simulink model "DYN_03x"  (R2021a)
settings: Solver=FixedStepAuto  StartTime=0.0  StopTime=10  FixedStep=0.001  RelTol=1e-3
(part 1 of 9)
settings Model: Creator=TMP  LastModifiedBy=TMP
settings SolverCC: AlgebraicLoopSolver=TrustRegion
settings DebuggingCC: SFMachineParentedDataDiag=warning

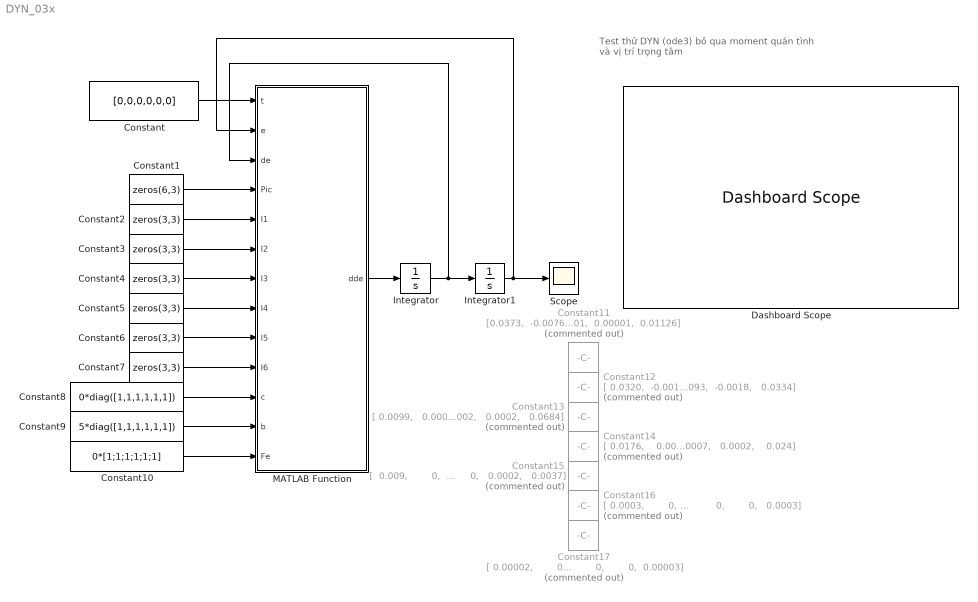
== system DYN_03x ==
  note: Test thử DYN (ode3)
      | bỏ qua moment quán tình và vị trí trọng tâm
  Constant : Constant  Value=[0,0,0,0,0,0]
  Constant1 : Constant  Value=zeros(6,3)
  Constant10 : Constant  Value=0*[1;1;1;1;1;1]
  Constant11 : Constant  Commented=on  Value=|
      | [0.0373,  -0.0076,   0.1064;
      |        0.1127,   0.0065,   0.0648;
      |        0.0447,   0.0125,  -0.0554;
      |        0.0006,   0.0052,   0.1068;
      |             0,   0.0062,   0.0195;
      |      -0.00001,  0.00001,  0.01126]
  Constant12 : Constant  Commented=on  Value=|
      | [ 0.0320,  -0.0017,   0.0093;
      |       -0.0017,   0.0364,  -0.0018;
      |        0.0093,  -0.0018,   0.0334]
  Constant13 : Constant  Commented=on  Value=|
      | [ 0.0099,   0.0008,  -0.0002;
      |        0.0008,   0.0646,   0.0002;
      |       -0.0002,   0.0002,   0.0684]
  Constant14 : Constant  Commented=on  Value=|
      | [ 0.0176,    0.001,   0.0007;
      |         0.001,   0.0195,   0.0002;
      |        0.0007,   0.0002,    0.024]
  Constant15 : Constant  Commented=on  Value=|
      | [  0.009,        0,        0;
      |             0,   0.0081,   0.0002;
      |             0,   0.0002,   0.0037]
  Constant16 : Constant  Commented=on  Value=|
      | [ 0.0003,        0,        0;
      |             0,   0.0002,        0;
      |             0,        0,   0.0003]
  Constant17 : Constant  Commented=on  Value=|
      | [ 0.00002,        0,        0;
      |              0,  0.00002,        0;
      |              0,        0,  0.00003]
  Constant{2..7} (6 alike) : Constant  Value=zeros(3,3)
  Constant8 : Constant  Value=0*diag([1,1,1,1,1,1])
  Constant9 : Constant  Value=5*diag([1,1,1,1,1,1])
  Dashboard Scope : DashboardScope
  Integrator : Integrator  InitialCondition=[0;0;0;0;0;0]
  Integrator1 : Integrator  InitialCondition=[0;0;0;0;0;0]
  MATLAB Function : MATLAB Function  TreatAsAtomicUnit=on
  Scope : Scope
  wires:
  MATLAB Function/1(dde) -> Integrator/1
  Integrator/1 -> MATLAB Function/3(de), Integrator1/1
  Integrator1/1 -> MATLAB Function/2(e), Scope/1
  Constant/1 -> MATLAB Function/1(t)
  Constant1/1 -> MATLAB Function/4(Pic)
  Constant2/1 -> MATLAB Function/5(I1)
  Constant3/1 -> MATLAB Function/6(I2)
  Constant4/1 -> MATLAB Function/7(I3)
  Constant5/1 -> MATLAB Function/8(I4)
  Constant6/1 -> MATLAB Function/9(I5)
  Constant7/1 -> MATLAB Function/10(I6)
  Constant8/1 -> MATLAB Function/11(c)
  Constant9/1 -> MATLAB Function/12(b)
  Constant10/1 -> MATLAB Function/13(Fe)
